simulink model "M1_P3_A_3"  (R2023a)
settings: Solver=VariableStepAuto  StartTime=0.0  StopTime=1.5  RelTol=1e-3
values from neighbouring files (symbols this model uses):
  f_eff = 0.001    [varMotor.mat]    (also in varMotor2.mat = 0.022)
  J_eff = 4e-05    [varMotor.mat]    (also in varMotor2.mat = 0.00025)
  Kb = 0.02    [varMotor.mat]    (also in varMotor2.mat = 0.041)
  Ktn = 0.026    [varMotor.mat]    (also in varMotor2.mat = 0.047)
  L = 0.062    [varMotor.mat]    (also in varMotor2.mat)
  R = 2.5    [varMotor.mat]    (also in varMotor2.mat)
settings Model: Creator=azzam  LastModifiedBy=azzam

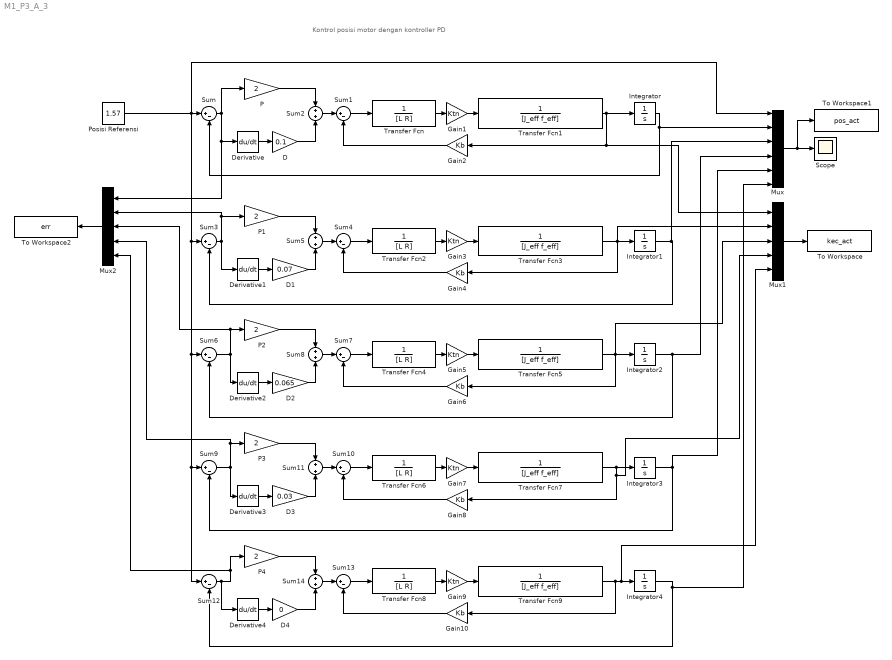
== system M1_P3_A_3 ==
  note: Kontrol posisi motor dengan kontroller PD
  D : Gain  Gain=0.1
  D1 : Gain  Gain=0.07
  D2 : Gain  Gain=0.065
  D3 : Gain  Gain=0.03
  D4 : Gain  Gain=0
  Derivative{,1..4} (5 alike) : Derivative
  Gain{1,3,5,7,9} (5 alike) : Gain  Gain=Ktn
  Gain{2,4,6,8,10} (5 alike) : Gain  Gain=Kb
  Integrator{,1..4} (5 alike) : Integrator
  Mux : Mux  Inputs=6
  Mux1 : Mux  Inputs=5
  Mux2 : Mux  Inputs=5
  P{,1..4} (5 alike) : Gain  Gain=2
  Posisi Referensi : Constant  Value=1.57
  Scope : Scope
  Sum{,1,3..4,6..7,9..10,12..13} (10 alike) : Sum  Inputs=|+-
  Sum{2,5,8,11,14} (5 alike) : Sum
  To Workspace : ToWorkspace  VariableName=kec_act  SaveFormat=Timeseries  SampleTime=-1
  To Workspace1 : ToWorkspace  VariableName=pos_act  SaveFormat=Timeseries  SampleTime=-1
  To Workspace2 : ToWorkspace  VariableName=err  SaveFormat=Timeseries  SampleTime=-1
  Transfer Fcn{,2,4,6,8} (5 alike) : TransferFcn  Denominator=[L R]
  Transfer Fcn{1,3,5,7,9} (5 alike) : TransferFcn  Denominator=[J_eff f_eff]
  wires:
  Derivative/1 -> D/1
  D/1 -> Sum2/2
  P/1 -> Sum2/1
  Sum/1 -> Derivative/1, Mux2/1, P/1
  Sum1/1 -> Transfer Fcn/1
  Mux/1 -> To Workspace1/1, Scope/1
  Gain2/1 -> Sum1/2
  Transfer Fcn1/1 -> Mux1/1, Gain2/1, Integrator/1
  Transfer Fcn/1 -> Gain1/1
  Gain1/1 -> Transfer Fcn1/1
  Sum2/1 -> Sum1/1
  Integrator/1 -> Sum/2, Mux/2
  Mux2/1 -> To Workspace2/1
  Mux1/1 -> To Workspace/1
  Transfer Fcn3/1 -> Gain4/1, Mux1/2, Integrator1/1
  Transfer Fcn2/1 -> Gain3/1
  Gain4/1 -> Sum4/2
  Sum5/1 -> Sum4/1
  Gain3/1 -> Transfer Fcn3/1
  Sum4/1 -> Transfer Fcn2/1
  P1/1 -> Sum5/1
  Integrator1/1 -> Mux/3, Sum3/2
  Derivative1/1 -> D1/1
  D1/1 -> Sum5/2
  Sum3/1 -> Derivative1/1, Mux2/2, P1/1
  Transfer Fcn5/1 -> Mux1/3, Gain6/1, Integrator2/1
  Transfer Fcn4/1 -> Gain5/1
  Gain6/1 -> Sum7/2
  Sum8/1 -> Sum7/1
  Gain5/1 -> Transfer Fcn5/1
  Sum7/1 -> Transfer Fcn4/1
  P2/1 -> Sum8/1
  Integrator2/1 -> Sum6/2, Mux/4
  Derivative2/1 -> D2/1
  D2/1 -> Sum8/2
  Sum6/1 -> Mux2/3, P2/1, Derivative2/1
  Transfer Fcn7/1 -> Mux1/4, Gain8/1, Integrator3/1
  Transfer Fcn6/1 -> Gain7/1
  Gain8/1 -> Sum10/2
  Sum11/1 -> Sum10/1
  Gain7/1 -> Transfer Fcn7/1
  Sum10/1 -> Transfer Fcn6/1
  P3/1 -> Sum11/1
  Integrator3/1 -> Mux/5, Sum9/2
  Derivative3/1 -> D3/1
  D3/1 -> Sum11/2
  Sum9/1 -> Derivative3/1, Mux2/4, P3/1
  Posisi Referensi/1 -> Sum12/1, Sum9/1, Sum6/1, Sum3/1, Mux/1, Sum/1
  Transfer Fcn9/1 -> Mux1/5, Integrator4/1, Gain10/1
  Transfer Fcn8/1 -> Gain9/1
  Gain10/1 -> Sum13/2
  Sum14/1 -> Sum13/1
  Gain9/1 -> Transfer Fcn9/1
  Sum13/1 -> Transfer Fcn8/1
  P4/1 -> Sum14/1
  Integrator4/1 -> Mux/6, Sum12/2
  Derivative4/1 -> D4/1
  D4/1 -> Sum14/2
  Sum12/1 -> Derivative4/1, Mux2/5, P4/1
